simulink subsystem "diff_int"  (R2022b)
settings: Solver=VariableStepAuto  StartTime=0.0  StopTime=10.0  RelTol=1e-3
settings Model: Creator=User  LastModifiedBy=User

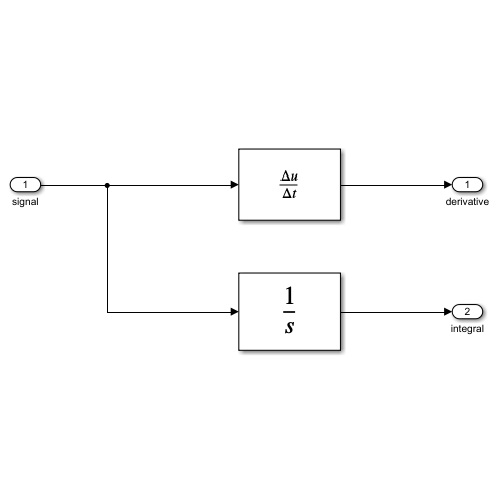
[thumbnail: Simulink's stored preview of the top-level diagram]
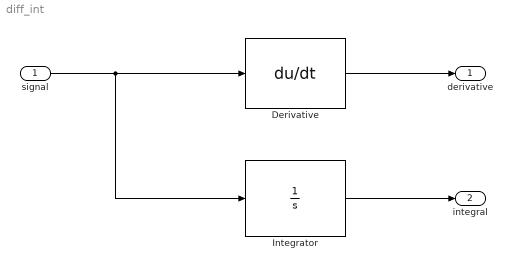
== system diff_int ==
  signal : Inport
  Derivative : Derivative
  Integrator : Integrator
  derivative : Outport
  integral : Outport  Port=2
  wires:
  Derivative/1 -> derivative/1
  Integrator/1 -> integral/1
  signal/1 -> Integrator/1, Derivative/1
